simulink model "robocup_model"  (Simulink 8.5)
settings: Solver=ode45  StartTime=0.0  StopTime=7  RelTol=1e-3
libraries: simulink x1
settings Model: Creator=justbuchanan  LastModifiedBy=Simon  CovSFcnEnable=off
settings DataIOCC: SignalLoggingSaveFormat=Dataset
settings OptimizationCC: BlockReduction=off  InlineParams=on  BufferReuse=off  ExpressionDepthLimit=128  SimCompilerOptimization=on
settings DebuggingCC: UnderspecifiedInitializationDetection=Simplified  MergeDetectMultiDrivingBlocksExec=error  SolverPrmCheckMsg=warning  FcnCallInpInsideContextMsg=EnableAllAsError  StateNameClashWarn=none
settings HardwareCC: ProdLargestAtomicInteger=Long  ProdLargestAtomicFloat=Double  ProdEndianess=LittleEndian  ProdHWDeviceType=ARM Compatible->ARM Cortex
settings GRTTargetCC: CombineOutputUpdateFcns=on  GRTInterface=off

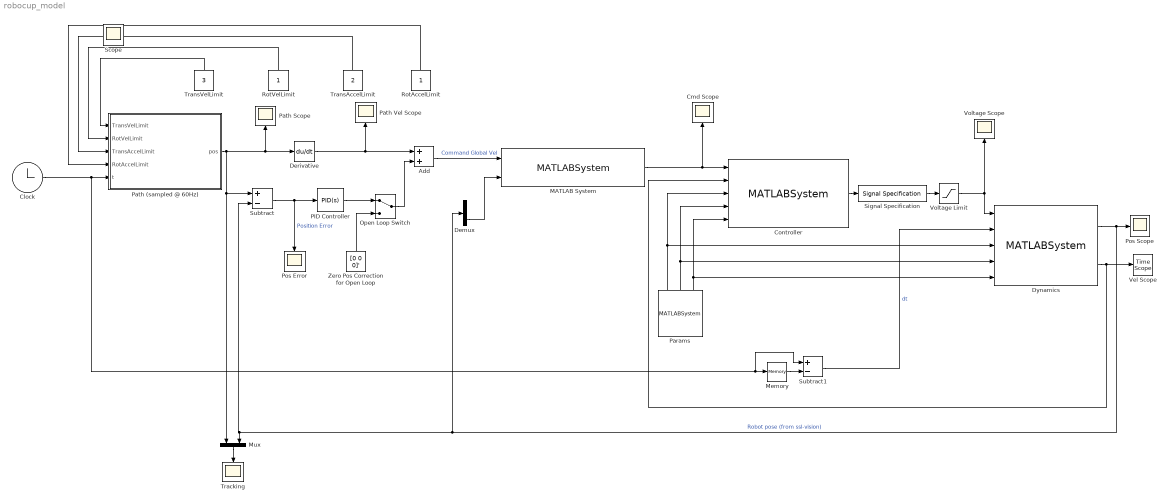
== system robocup_model ==
  Add : Sum
  Clock : Clock
  Cmd Scope : Scope
      settings: SaveName=ScopeData4
  Controller : MATLABSystem  System=RobotLqr  trans_vel_weight=5  rot_vel_weight=0.1  u_weight=1  SimulateUsing=Interpreted execution
      mask Type: RobotLqr
      mask Display:
      | disp('RobotLqr');
      | port_label('input',1,'Cmd Velocity');
      | port_label('input',2,'Curr. Velocity');
      | port_label('input',3,'A_1');
      | port_label('input',4,'A_2');
      | port_label('input',5,'B');
      | port_label('output',1,'u');
  Demux : Demux  Outputs=3
  Derivative : Derivative
  Dynamics : MATLABSystem  System=Robot  SimulateUsing=Interpreted execution
      mask Type: Robot
      mask Display:
      | disp(['RoboCup Robot' char(10) 'Dynamics']);
      | port_label('input',1,'Motor Voltages');
      | port_label('input',2,'dt');
      | port_label('input',3,'A_1');
      | port_label('input',4,'A_2');
      | port_label('input',5,'B');
      | port_label('output',1,'Robot pose');
      | port_label('output',2,'Robot velocity');
  MATLAB System : MATLABSystem  System=Global2Body  SimulateUsing=Code generation
      mask Type: Global2Body
      mask Display:
      | disp('Global2Body');
      | port_label('input',1,'Global Velocity');
      | port_label('input',2,'Robot angle');
      | port_label('output',1,'Body Velocity');
  Memory : Memory  X0=-0.1
  Mux : Mux  Inputs=2
  Open Loop Switch : ManualSwitch
  PID Controller : simulink/Continuous/PID Controller  Controller=PID  TimeDomain=Continuous-time  SampleTime=-1  IntegratorMethod=Forward Euler  FilterMethod=Forward Euler  Form=Parallel  UseFilter=on  ControllerParametersSource=internal  P=4  I=0  D=0  N=100  InitialConditionSource=internal  InitialConditionForIntegrator=0  InitialConditionForFilter=0  ExternalReset=none  LimitOutput=off  UpperSaturationLimit=inf  LowerSaturationLimit=-inf  LinearizeAsGain=on  AntiWindupMode=none  Kb=1  TrackingMode=off  Kt=1  PParamMin=[]  PParamMax=[]  IParamMin=[]  IParamMax=[]  DParamMin=[]  DParamMax=[]  NParamMin=[]  NParamMax=[]  KbParamMin=[]  KbParamMax=[]  KtParamMin=[]  KtParamMax=[]  POutMin=[]  POutMax=[]  IOutMin=[]  IOutMax=[]  DOutMin=[]  DOutMax=[]  NOutMin=[]  NOutMax=[]  KbOutMin=[]  KbOutMax=[]  KtOutMin=[]  KtOutMax=[]  IntegratorOutMin=[]  IntegratorOutMax=[]  FilterOutMin=[]  FilterOutMax=[]  SumOutMin=[]  SumOutMax=[]  SumI1OutMin=[]  SumI1OutMax=[]  SumI2OutMin=[]  SumI2OutMax=[]  SumI3OutMin=[]  SumI3OutMax=[]  SumDOutMin=[]  SumDOutMax=[]  SaturationOutMin=[]  SaturationOutMax=[]  IntegratorContinuousStateAttributes=''  IntegratorStateMustResolveToSignalObject=off  IntegratorRTWStateStorageClass=Auto  FilterContinuousStateAttributes=''  FilterStateMustResolveToSignalObject=off  FilterRTWStateStorageClass=Auto  DifferentiatorICPrevScaledInput=0  DifferentiatorOutMin=[]  DifferentiatorOutMax=[]
  Params : MATLABSystem  System=RobotParams  M_bot=2.205  I_bot=0.00745879949  g=2.0/7.0  r=0.0285623  L=0.0798576  Rt=0.464  K_e=30.0/(380*pi)  K_t=0.0251  K_f=0.0001  I_asm=2.43695253e-5  V=18  wheel_angles=[38*pi/180.0, 142*pi/180.0, 225*pi/180.0, 315*pi/180.0]'  SimulateUsing=Code generation
      mask Type: RobotParams
      mask Display:
      | disp('RobotParams');
      | port_label('output',1,'A_1');
      | port_label('output',2,'A_2');
      | port_label('output',3,'B');
  Path (sampled @ 60Hz) : MATLAB Function  TreatAsAtomicUnit=on  SystemSampleTime=1/60
  Path Scope : Scope
      settings: SaveName=ScopeData5
  Path Vel Scope : Scope
      settings: SaveName=ScopeData6
  Pos Error : Scope
      settings: SaveName=ScopeData7
  Pos Scope : Scope
      settings: SaveName=ScopeData2
  RotAccelLimit : Constant
  RotVelLimit : Constant
  Signal Specification : SignalSpecification  OutDataTypeStr=double  Dimensions=[4 1]
  Subtract : Sum  Inputs=+-
  Subtract1 : Sum  Inputs=+-
  Tracking : Scope
      settings: YMin=-5.5  YMax=5.5  SaveName=ScopeData8
  TransAccelLimit : Constant  Value=2
  TransVelLimit : Constant  Value=3
  Vel Scope : TimeScope
  Voltage Limit : Saturate  UpperLimit=18  LowerLimit=-18
  Voltage Scope : Scope
      settings: SaveName=ScopeData3
  Zero Pos Correction for Open Loop : Constant  Value=[0 0 0]'
  Scope : Scope
  wires:
  Derivative/1 -> Add/1, Path Vel Scope/1
  Path (sampled @ 60Hz)/1(pos) -> Path Scope/1, Derivative/1, Subtract/1, Mux/1
  Subtract/1 -> PID Controller/1, Pos Error/1  "Position Error"
  Add/1 -> MATLAB System/1  "Command Global Vel"
  Subtract1/1 -> Dynamics/2  "dt"
  Params/1 -> Controller/3, Dynamics/3
  Params/2 -> Controller/4, Dynamics/4
  Params/3 -> Controller/5, Dynamics/5
  Dynamics/1 -> Pos Scope/1, Demux/1, Subtract/2, Mux/2  "Robot pose (from ssl-vision)"
  Dynamics/2 -> Vel Scope/1, Controller/2
  TransVelLimit/1 -> Path (sampled @ 60Hz)/1(TransVelLimit)
  RotVelLimit/1 -> Path (sampled @ 60Hz)/2(RotVelLimit)
  TransAccelLimit/1 -> Path (sampled @ 60Hz)/3(TransAccelLimit)
  RotAccelLimit/1 -> Path (sampled @ 60Hz)/4(RotAccelLimit)
  Controller/1 -> Signal Specification/1
  Clock/1 -> Subtract1/1, Memory/1, Path (sampled @ 60Hz)/5(t)
  Memory/1 -> Subtract1/2
  Open Loop Switch/1 -> Add/2
  PID Controller/1 -> Open Loop Switch/1
  Zero Pos Correction for Open Loop/1 -> Open Loop Switch/2
  Signal Specification/1 -> Voltage Limit/1
  Mux/1 -> Tracking/1
  Voltage Limit/1 -> Voltage Scope/1, Dynamics/1
  MATLAB System/1 -> Controller/1, Cmd Scope/1
  Demux/3 -> MATLAB System/2

== matlab function Path (sampled @ 60Hz) ==
  data: TransVelLimit input double; RotVelLimit input double; TransAccelLimit input double; RotAccelLimit input double; pos output double; t input double
function pos = path(TransVelLimit, RotVelLimit, TransAccelLimit, RotAccelLimit, t)
%#codegen

pos = [0 0 0]';

accel = [-1 1 0.9]';


rampTime = TransVelLimit/TransAccelLimit;
flatTime = 2;


% ramp-up
pos = pos + 0.5*accel*min(t,rampTime)^2;

% const speed
if t > rampTime
    vel = accel*rampTime;
    pos = pos + min(t-rampTime, flatTime)*vel;
end

% ramp-down
if t > rampTime + flatTime
    vi = accel*rampTime;
    rampDownT = min(t-rampTime-flatTime, rampTime);
    pos = pos + -0.5*accel*rampDownT^2 + vi*rampDownT;
end
